simulink model "MC_CVCR_rev6_sim_withc_code_S_function_contplant"  (R2017a)
settings: Solver=VariableStepAuto  StartTime=0.0  StopTime=0.1  FixedStep=T_sim  MaxStep=T_s/10  RelTol=1e-3  EnableMultiTasking=on
model workspace: external: MAT-File C:\Users\Gene\GoogleDrive\UW\Research\Simulation\Discrete CVCR\MATLAB\ws.mat (data not in the file)
values from neighbouring files (symbols this model uses):
  b_a = (-za1*zb1*zc1+1)*J_p/(T_s)    [MC_CVCR_rev6_code_withc_code_S_function.m]
  b_p = 1e-4    (= 0.0001)    [MC_CVCR_rev6_code_withc_code_S_function.m]
  J_p = 6.09e-5    (= 6.09e-05)    [MC_CVCR_rev6_code_withc_code_S_function.m]
  K_i = 2*pi*BW_CVCR*R_s    (= 183.719331443)    [MC_CVCR_rev6_code_withc_code_S_function.m]
  K_isa = ((-(za1+zb1+zc1)+3)*J_p-T_s*b_a-(T_s)^2*K_sa)/((T_s)^3)    [MC_CVCR_rev6_code_withc_code_S_function.m]
  K_p = 2*pi*BW_CVCR*L_s    (= 0.0699004365424)    [MC_CVCR_rev6_code_withc_code_S_function.m]
  K_sa = ((-(za1*zb1+za1*zc1+zb1*zc1)+3)*J_p-2*T_s*b_a)/((T_s)^2)    [MC_CVCR_rev6_code_withc_code_S_function.m]
  K_T = 3/2*K_e    (= 0.013078435501)    [MC_CVCR_rev6_code_withc_code_S_function.m]
  Ksf1 = 1000    [MC_CVCR_rev6_code_withc_code_S_function.m]
  Ksf2 = 4000    [MC_CVCR_rev6_code_withc_code_S_function.m]
  L_ds = 42.28e-6    (= 4.228e-05)    [MC_CVCR_rev6_code_withc_code_S_function.m]
  L_qs = 46.71e-6    (= 4.671e-05)    [MC_CVCR_rev6_code_withc_code_S_function.m]
  Lambda_pm = K_e/(P/2)    (= 0.00217973925016)    [MC_CVCR_rev6_code_withc_code_S_function.m]
  NegSpeedLimit = -600    [MC_CVCR_rev6_code_withc_code_S_function.m]
  P = 8    [MC_CVCR_rev6_code_withc_code_S_function.m]
  PosSpeedLimit = 600    [MC_CVCR_rev6_code_withc_code_S_function.m]
  R_s = 0.116959358962624    (= 0.116959358963)    [MC_CVCR_rev6_code_withc_code_S_function.m]
  T_s = 1/f_s    (= 5e-05)    [MC_CVCR_rev6_code_withc_code_S_function.m]
  T_u = 0.047    [MC_CVCR_rev6_code_withc_code_S_function.m]
libraries: dspsrcs4 x5
settings Model: Creator=Gene  LastModifiedBy=Gene
settings DataIOCC: SaveFormat=StructureWithTime
settings OptimizationCC: LifeSpan=inf
settings DebuggingCC: SFUnexpectedBacktrackingDiag=warning  SFNoUnconditionalDefaultTransitionDiag=warning  SFExecutionAtInitializationDiag=none
settings GRTTargetCC: TargetLangStandard=C89/C90 (ANSI)  GeneratePreprocessorConditionals=Disable all
settings ConfigComp: CovMetricSettings=dw  CovHtmlReporting=on  CovSaveCumulativeToWorkspaceVar=on  CovSaveSingleToWorkspaceVar=on  CovExternalEMLEnable=off

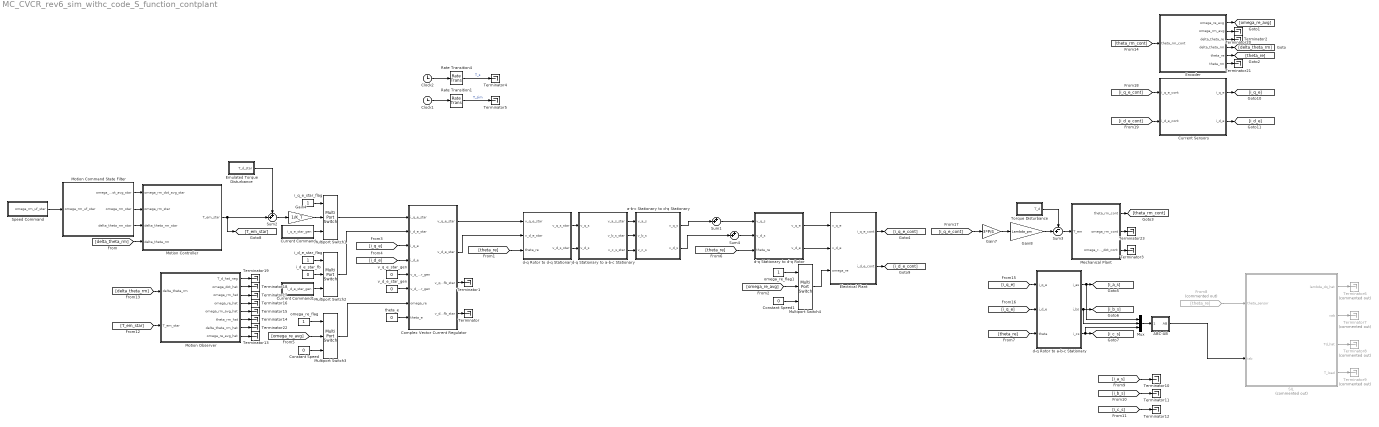
== system MC_CVCR_rev6_sim_withc_code_S_function_contplant ==
  ABC-AB : Subsystem
  Clock1 : Clock
  Clock2 : Clock
  Complex Vector Current Regulator : Subsystem
  Constant Speed : Constant  Value=0  SampleTime=-1
  Constant Speed1 : Constant  Value=0  SampleTime=-1
  Current Command : Subsystem
  Current Command1 : Subsystem
  Current Sensors : Subsystem  TreatAsAtomicUnit=on  SystemSampleTime=T_s
  Electrical Plant : Subsystem
  Emulated Torque Disturbance : Subsystem
  Encoder : Subsystem  TreatAsAtomicUnit=on  SystemSampleTime=T_s
  From8 : From  Commented=on  GotoTag=theta_re
  Gain4 : Gain  Gain=1/K_T
  Gain7 : Gain  Gain=3*P/4
  Gain8 : Gain  Gain=Lambda_pm
  Mechanical Plant : Subsystem
  Motion Command State Filter : Subsystem
  Motion Controller : Subsystem
  Motion Observer : Subsystem
  Multiport Switch{1..4} (4 alike) : MultiPortSwitch  Inputs=2
  Mux : Mux  Inputs=3
  Rate Transition1 : RateTransition  OutPortSampleTime=T_sim
  Rate Transition4 : RateTransition  OutPortSampleTime=T_s
  SIL : Subsystem  Commented=on  TreatAsAtomicUnit=on
  Speed Command : Subsystem
  Sum1 : Sum  Inputs=++|
  Sum2 : Sum  Inputs=++|
  Sum3 : Sum  Inputs=-+|
  Sum4 : Sum  Inputs=++|
  Terminator{,1..5,10..23} (20 alike) : Terminator
  Terminator{6..9} (4 alike) : Terminator  Commented=on
  Torque Disturbance : Subsystem
  a-b-c Stationary to d-q Stationary : Subsystem
  d-q Rotor to d-q Stationary : Subsystem
  d-q Rotor to a-b-c Stationary : Subsystem  TreatAsAtomicUnit=on  SystemSampleTime=T_s
  d-q Stationary to a-b-c Stationary : Subsystem
  d-q Stationary to d-q Rotor : Subsystem
  i_d_e_star_fb : Constant  Value=0  SampleTime=-1
  i_d_e_star_flag : Constant  SampleTime=-1
  i_q_e_star_flag : Constant  SampleTime=-1
  omega_re_flag : Constant  SampleTime=-1
  omega_re_flag1 : Constant  SampleTime=-1
  theta_e : Constant  Value=0
  v_d_e_star_gen : Constant  Value=0
  v_q_e_star_gen : Constant  Value=0
  wires:
  Multiport Switch2/1 -> Complex Vector Current Regulator/2(i_d_e_star)
  Gain4/1 -> Multiport Switch1/2
  Complex Vector Current Regulator/4(v_d_e_sfb_star) -> Terminator/1
  Complex Vector Current Regulator/3(v_q_e_sfb_star) -> Terminator1/1
  v_d_e_star_gen/1 -> Complex Vector Current Regulator/6(v_d_e_star_gen)
  v_q_e_star_gen/1 -> Complex Vector Current Regulator/5(v_q_e_star_gen)
  theta_e/1 -> Complex Vector Current Regulator/8(theta_e)
  Sum2/1 -> Gain4/1
  d-q Stationary to d-q Rotor/1(v_q_e) -> Electrical Plant/1(v_q_e)
  d-q Stationary to d-q Rotor/2(v_d_e) -> Electrical Plant/2(v_d_e)
  Gain7/1 -> Gain8/1
  Gain8/1 -> Sum3/2
  Sum3/1 -> Mechanical Plant/1(T_em)
  Torque Disturbance/1(T_d) -> Sum3/1
  Speed Command/1(omega_rm_uf_star) -> Motion Command State Filter/1(omega_rm_uf_star)
  Emulated Torque Disturbance/1(T_d_star) -> Sum2/1
  Motion Command State Filter/1(omega_rm_dot_avg_star) -> Motion Controller/1(omega_rm_dot_avg_star)
  Motion Command State Filter/2(omega_rm_star) -> Motion Controller/2(omega_rm_star)
  Motion Command State Filter/3(delta_theta_rm_star) -> Motion Controller/3(delta_theta_rm_star)
  Motion Controller/1(T_em_star) -> Sum2/2, [T_em_star]
  [delta_theta_rm] -> Motion Controller/4(delta_theta_rm)
  Multiport Switch4/1 -> Electrical Plant/3(omega_re)
  Multiport Switch3/1 -> Complex Vector Current Regulator/7(omega_re)
  [i_q_e] -> Complex Vector Current Regulator/3(i_q_e)
  [i_d_e] -> Complex Vector Current Regulator/4(i_d_e)
  Clock2/1 -> Rate Transition4/1
  Rate Transition4/1 -> Terminator4/1  "T_s"
  Rate Transition1/1 -> Terminator5/1  "T_sim"
  Clock1/1 -> Rate Transition1/1
  Current Command/1(i_q_e_star_gen) -> Multiport Switch1/3
  i_q_e_star_flag/1 -> Multiport Switch1/1
  Multiport Switch1/1 -> Complex Vector Current Regulator/1(i_q_e_star)
  i_d_e_star_fb/1 -> Multiport Switch2/2
  Current Command1/1(i_d_e_star_gen) -> Multiport Switch2/3
  i_d_e_star_flag/1 -> Multiport Switch2/1
  Constant Speed/1 -> Multiport Switch3/3
  [omega_re_avg] -> Multiport Switch3/2
  omega_re_flag/1 -> Multiport Switch3/1
  Constant Speed1/1 -> Multiport Switch4/3
  omega_re_flag1/1 -> Multiport Switch4/1
  [omega_re_avg] -> Multiport Switch4/2
  d-q Rotor to d-q Stationary/1(v_q_s_star) -> d-q Stationary to a-b-c Stationary/1(v_q_s)
  d-q Rotor to d-q Stationary/2(v_d_s_star) -> d-q Stationary to a-b-c Stationary/2(v_d_s)
  Sum1/1 -> d-q Stationary to d-q Rotor/1(v_q_s)
  Sum4/1 -> d-q Stationary to d-q Rotor/2(v_d_s)
  d-q Stationary to a-b-c Stationary/1(v_a_s_star) -> a-b-c Stationary to d-q Stationary/1(v_a_s)
  d-q Stationary to a-b-c Stationary/2(v_b_s_star) -> a-b-c Stationary to d-q Stationary/2(v_b_s)
  d-q Stationary to a-b-c Stationary/3(v_c_s_star) -> a-b-c Stationary to d-q Stationary/3(v_c_s)
  [theta_re] -> d-q Rotor to d-q Stationary/3(theta_re)
  [theta_re] -> d-q Stationary to d-q Rotor/3(theta_re)
  Complex Vector Current Regulator/2(v_d_e_star) -> d-q Rotor to d-q Stationary/2(v_d_e_star)
  Complex Vector Current Regulator/1(v_q_e_star) -> d-q Rotor to d-q Stationary/1(v_q_e_star)
  [theta_re] -> d-q Rotor to a-b-c Stationary/3(theta)
  Mux/1 -> ABC-AB/1(ABC)
  d-q Rotor to a-b-c Stationary/3(i_cs) -> Mux/3, [i_c_s]
  d-q Rotor to a-b-c Stationary/2(i_bs) -> Mux/2, [i_b_s]
  d-q Rotor to a-b-c Stationary/1(i_as) -> Mux/1, [i_a_s]
  From8/1 -> SIL/1(theta_sensor)
  ABC-AB/1(AB) -> SIL/2(iab)
  SIL/1(lambda_dq_hat) -> Terminator6/1
  SIL/2(vab) -> Terminator7/1
  SIL/3(Td_hat) -> Terminator8/1
  SIL/4(T_load) -> Terminator9/1
  [i_a_s] -> Terminator10/1
  [i_b_s] -> Terminator11/1
  [i_c_s] -> Terminator12/1
  [delta_theta_rm] -> Motion Observer/1(delta_theta_rm)
  [T_em_star] -> Motion Observer/2(T_em_star)
  Motion Observer/7(delta_theta_rm_hat) -> Terminator22/1
  Motion Observer/6(theta_rm_hat) -> Terminator14/1
  Motion Observer/5(omega_rm_avg_hat) -> Terminator15/1
  Motion Observer/4(omega_re_hat) -> Terminator16/1
  Motion Observer/3(omega_rm_hat) -> Terminator17/1
  Motion Observer/2(omega_dot_hat) -> Terminator18/1
  Motion Observer/1(T_d_hat_neg) -> Terminator19/1
  Motion Observer/8(omega_re_avg_hat) -> Terminator13/1
  a-b-c Stationary to d-q Stationary/1(v_q_s) -> Sum1/2
  a-b-c Stationary to d-q Stationary/2(v_d_s) -> Sum4/2
  [i_q_e] -> d-q Rotor to a-b-c Stationary/2(i_d_e)
  Encoder/4(delta_theta_rm) -> [delta_theta_rm]
  Encoder/2(omega_rm_avg) -> Terminator20/1
  Encoder/6(theta_rm) -> Terminator21/1
  Encoder/1(omega_re_avg) -> [omega_re_avg]
  Encoder/5(theta_re) -> [theta_re]
  Encoder/3(delta_theta_re) -> Terminator2/1
  Mechanical Plant/3(omega_rm_dot_cont) -> Terminator3/1
  Mechanical Plant/2(omega_rm_cont) -> Terminator23/1
  Mechanical Plant/1(theta_rm_cont) -> [theta_rm_cont]
  [theta_rm_cont] -> Encoder/1(theta_rm_cont)
  Electrical Plant/2(i_d_e_cont) -> [i_d_e_cont]
  Electrical Plant/1(i_q_e_cont) -> [i_q_e_cont]
  [i_q_e] -> d-q Rotor to a-b-c Stationary/1(i_q_e)
  [i_q_e_cont] -> Gain7/1
  [i_d_e_cont] -> Current Sensors/2(i_d_e_cont)
  [i_q_e_cont] -> Current Sensors/1(i_q_e_cont)
  Current Sensors/1(i_q_e) -> [i_q_e]
  Current Sensors/2(i_d_e) -> [i_d_e]

== system MC_CVCR_rev6_sim_withc_code_S_function_contplant/ABC-AB ==
  ABC : Inport
  Mux2 : Mux  Inputs=2
  a : Fcn  Expr=2/3*(u[1] -0.5*u[2] - 0.5*u[3])
  b : Fcn  Expr=2/3*(0 +sqrt(3)/2*u[2] - sqrt(3)/2*u[3])
  AB : Outport
  wires:
  Mux2/1 -> AB/1
  b/1 -> Mux2/2
  ABC/1 -> b/1, a/1
  a/1 -> Mux2/1

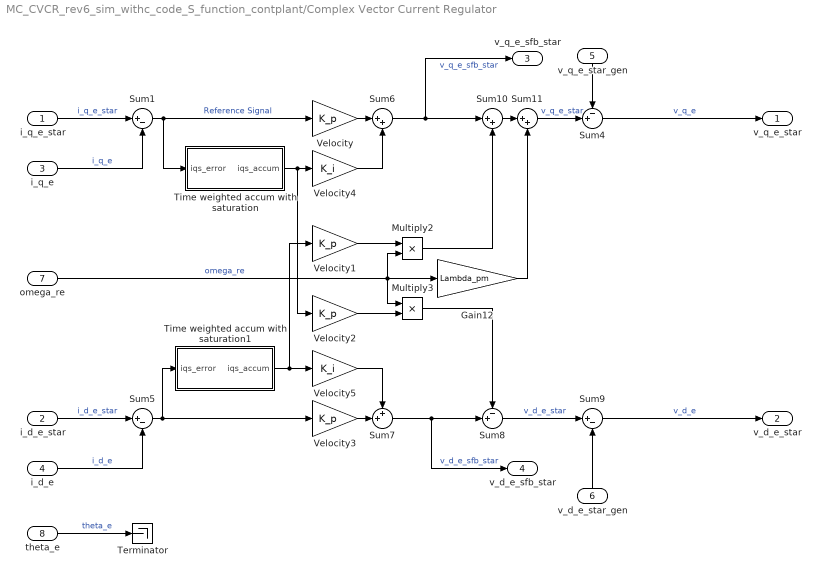
== system MC_CVCR_rev6_sim_withc_code_S_function_contplant/Complex Vector Current Regulator ==
  i_q_e_star : Inport
  i_d_e_star : Inport  Port=2
  i_q_e : Inport  Port=3
  i_d_e : Inport  Port=4
  v_q_e_star_gen : Inport  Port=5
  v_d_e_star_gen : Inport  Port=6
  omega_re : Inport  Port=7
  theta_e : Inport  Port=8
  Gain12 : Gain  Gain=Lambda_pm
  Multiply2 : Product  Inputs=**
  Multiply3 : Product  Inputs=**
  Sum1 : Sum  Priority=1  Inputs=|+-
  Sum10 : Sum  Priority=1  Inputs=|++
  Sum11 : Sum  Priority=1  Inputs=|++
  Sum4 : Sum  Priority=1  Inputs=-+|
  Sum5 : Sum  Priority=1  Inputs=|+-
  Sum6 : Sum  Priority=1  Inputs=|++
  Sum7 : Sum  Priority=1  Inputs=++|
  Sum8 : Sum  Priority=1  Inputs=-+|
  Sum9 : Sum  Inputs=|+-
  Terminator : Terminator
  Time weighted accum with saturation : Subsystem
  Time weighted accum with saturation1 : Subsystem
  Velocity{,1..3} (4 alike) : Gain  Gain=K_p  SampleTime=T_s
  Velocity4 : Gain  Gain=K_i  SampleTime=T_s
  Velocity5 : Gain  Gain=K_i  SampleTime=T_s
  v_q_e_star : Outport
  v_d_e_star : Outport  Port=2
  v_q_e_sfb_star : Outport  Port=3
  v_d_e_sfb_star : Outport  Port=4
  wires:
  Velocity2/1 -> Multiply3/2
  Sum1/1 -> Velocity/1, Time weighted accum with saturation/1(iqs_error)  "Reference Signal"
  i_q_e_star/1 -> Sum1/1  "i_q_e_star"
  i_d_e_star/1 -> Sum5/1  "i_d_e_star"
  Time weighted accum with saturation/1(iqs_accum) -> Velocity4/1, Velocity2/1
  Sum5/1 -> Time weighted accum with saturation1/1(iqs_error), Velocity3/1
  Time weighted accum with saturation1/1(iqs_accum) -> Velocity5/1, Velocity1/1
  Velocity4/1 -> Sum6/2
  Velocity/1 -> Sum6/1
  Velocity3/1 -> Sum7/2
  Velocity5/1 -> Sum7/1
  Sum7/1 -> v_d_e_sfb_star/1, Sum8/2  "v_d_e_sfb_star"
  Sum6/1 -> v_q_e_sfb_star/1, Sum10/1  "v_q_e_sfb_star"
  Multiply3/1 -> Sum8/1
  Multiply2/1 -> Sum10/2
  Sum11/1 -> Sum4/2  "v_q_e_star"
  Sum10/1 -> Sum11/1
  Gain12/1 -> Sum11/2
  Sum8/1 -> Sum9/1  "v_d_e_star"
  v_q_e_star_gen/1 -> Sum4/1
  Velocity1/1 -> Multiply2/1
  omega_re/1 -> Multiply3/1, Gain12/1, Multiply2/2  "omega_re"
  v_d_e_star_gen/1 -> Sum9/2
  theta_e/1 -> Terminator/1  "theta_e"
  Sum4/1 -> v_q_e_star/1  "v_q_e"
  Sum9/1 -> v_d_e_star/1  "v_d_e"
  i_q_e/1 -> Sum1/2  "i_q_e"
  i_d_e/1 -> Sum5/2  "i_d_e"

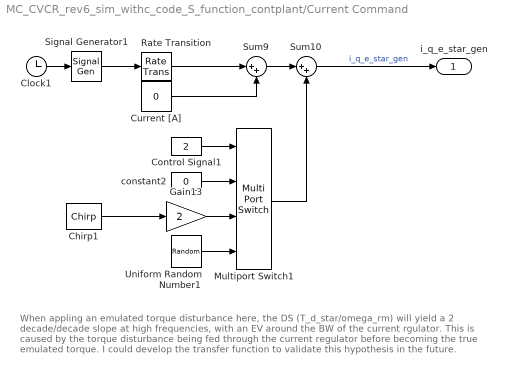
== system MC_CVCR_rev6_sim_withc_code_S_function_contplant/Current Command ==
  note: When appling an emulated torque disturbance here, the DS (T_d_star/omega_rm) will yield
      | a 2 decade/decade slope at high frequencies, with an EV around the BW of the current rgulator.
      | This is caused by the torque disturbance being fed through the current regulator before becoming the true emulated torque.
      |
      | I could develop the transfer function to validate this hypothesis in the future.
  Chirp1 : dspsrcs4/Chirp  sweep=Logarithmic  mode=Bidirectional  f0=0.1  f1=1000  t1=2  Tsweep=2  phase=0  Ts=T_s  spf=1  datatype=Double  OutputFrames=on
      settings: SourceProductName=DSP System Toolbox
  Clock1 : Clock
  Control Signal1 : Constant  Value=2
  Current [A] : Constant  Value=0
  Gain13 : Gain  Gain=2
  Multiport Switch1 : MultiPortSwitch
  Rate Transition : RateTransition  OutPortSampleTime=T_s
  Signal Generator1 : SignalGenerator  TimeSource=Use external signal  Amplitude=0
  Sum10 : Sum  Inputs=|++
  Sum9 : Sum  Inputs=|++
  Uniform Random Number1 : UniformRandomNumber  Minimum=-0.1  Maximum=0.1  SampleTime=T_s
  constant2 : Constant  Value=0
  i_q_e_star_gen : Outport
  wires:
  Multiport Switch1/1 -> Sum10/2
  Chirp1/1 -> Gain13/1
  Uniform Random Number1/1 -> Multiport Switch1/4
  Current [A]/1 -> Sum9/2
  Signal Generator1/1 -> Rate Transition/1
  Control Signal1/1 -> Multiport Switch1/1
  Clock1/1 -> Signal Generator1/1
  constant2/1 -> Multiport Switch1/2
  Sum9/1 -> Sum10/1
  Gain13/1 -> Multiport Switch1/3
  Sum10/1 -> i_q_e_star_gen/1  "i_q_e_star_gen"
  Rate Transition/1 -> Sum9/1

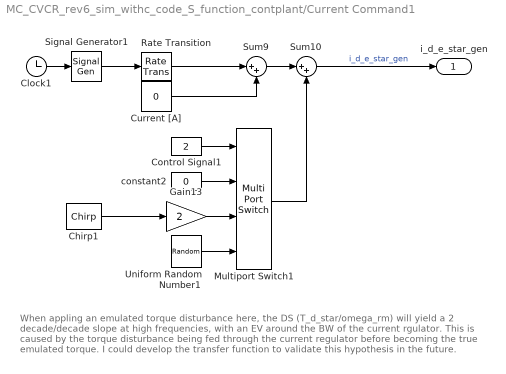
== system MC_CVCR_rev6_sim_withc_code_S_function_contplant/Current Command1 ==
  note: When appling an emulated torque disturbance here, the DS (T_d_star/omega_rm) will yield
      | a 2 decade/decade slope at high frequencies, with an EV around the BW of the current rgulator.
      | This is caused by the torque disturbance being fed through the current regulator before becoming the true emulated torque.
      |
      | I could develop the transfer function to validate this hypothesis in the future.
  Chirp1 : dspsrcs4/Chirp  sweep=Logarithmic  mode=Bidirectional  f0=0.1  f1=1000  t1=2  Tsweep=2  phase=0  Ts=T_s  spf=1  datatype=Double  OutputFrames=on
      settings: SourceProductName=DSP System Toolbox
  Clock1 : Clock
  Control Signal1 : Constant  Value=2
  Current [A] : Constant  Value=0
  Gain13 : Gain  Gain=2
  Multiport Switch1 : MultiPortSwitch
  Rate Transition : RateTransition  OutPortSampleTime=T_s
  Signal Generator1 : SignalGenerator  TimeSource=Use external signal  Amplitude=0
  Sum10 : Sum  Inputs=|++
  Sum9 : Sum  Inputs=|++
  Uniform Random Number1 : UniformRandomNumber  Minimum=-0.1  Maximum=0.1  SampleTime=T_s
  constant2 : Constant  Value=0
  i_d_e_star_gen : Outport
  wires:
  Multiport Switch1/1 -> Sum10/2
  Chirp1/1 -> Gain13/1
  Uniform Random Number1/1 -> Multiport Switch1/4
  Current [A]/1 -> Sum9/2
  Signal Generator1/1 -> Rate Transition/1
  Control Signal1/1 -> Multiport Switch1/1
  Clock1/1 -> Signal Generator1/1
  constant2/1 -> Multiport Switch1/2
  Sum9/1 -> Sum10/1
  Gain13/1 -> Multiport Switch1/3
  Sum10/1 -> i_d_e_star_gen/1  "i_d_e_star_gen"
  Rate Transition/1 -> Sum9/1

== system MC_CVCR_rev6_sim_withc_code_S_function_contplant/Current Sensors ==
  i_q_e_cont : Inport
  i_d_e_cont : Inport  Port=2
  i_q_e : Outport
  i_d_e : Outport  Port=2
  wires:
  i_q_e_cont/1 -> i_q_e/1  "i_q_e"
  i_d_e_cont/1 -> i_d_e/1  "i_q_e"

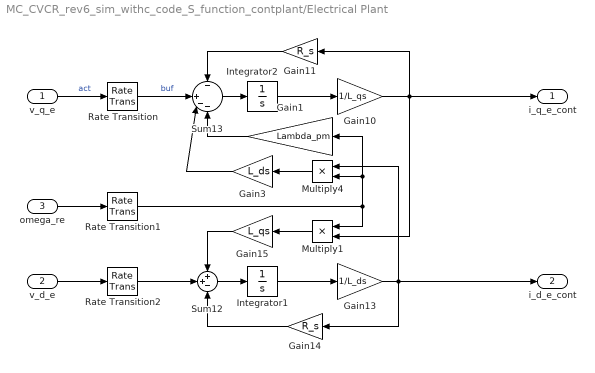
== system MC_CVCR_rev6_sim_withc_code_S_function_contplant/Electrical Plant ==
  v_q_e : Inport
  v_d_e : Inport  Port=2
  omega_re : Inport  Port=3
  Gain1 : Gain  Gain=Lambda_pm
  Gain10 : Gain  Gain=1/L_qs
  Gain11 : Gain  Gain=R_s
  Gain13 : Gain  Gain=1/L_ds
  Gain14 : Gain  Gain=R_s
  Gain15 : Gain  Gain=L_qs
  Gain3 : Gain  Gain=L_ds
  Integrator1 : Integrator
  Integrator2 : Integrator
  Multiply1 : Product  Inputs=**
  Multiply4 : Product  Inputs=**
  Rate Transition : RateTransition
  Rate Transition1 : RateTransition
  Rate Transition2 : RateTransition
  Sum12 : Sum  Inputs=++-
  Sum13 : Sum  Inputs=-|+--
  i_q_e_cont : Outport
  i_d_e_cont : Outport  Port=2
  wires:
  v_d_e/1 -> Rate Transition2/1
  v_q_e/1 -> Rate Transition/1  "act"
  Integrator1/1 -> Gain13/1
  Gain13/1 -> i_d_e_cont/1, Gain14/1, Multiply4/1
  Sum12/1 -> Integrator1/1
  Integrator2/1 -> Gain10/1
  Gain10/1 -> Multiply1/2, i_q_e_cont/1, Gain11/1
  Sum13/1 -> Integrator2/1
  Gain3/1 -> Sum13/3
  Gain15/1 -> Sum12/1
  Gain14/1 -> Sum12/3
  Gain11/1 -> Sum13/1
  Multiply1/1 -> Gain15/1
  Multiply4/1 -> Gain3/1
  omega_re/1 -> Rate Transition1/1
  Gain1/1 -> Sum13/4
  Rate Transition/1 -> Sum13/2  "buf"
  Rate Transition1/1 -> Multiply1/1, Gain1/1, Multiply4/2
  Rate Transition2/1 -> Sum12/2

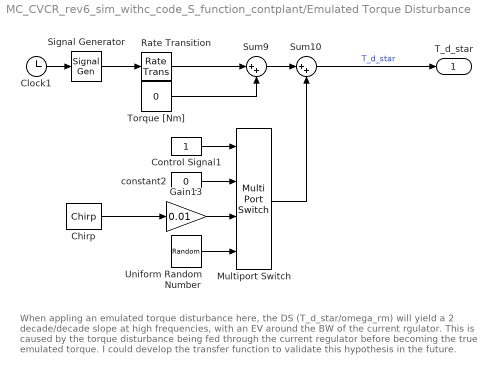
== system MC_CVCR_rev6_sim_withc_code_S_function_contplant/Emulated Torque Disturbance ==
  note: When appling an emulated torque disturbance here, the DS (T_d_star/omega_rm) will yield
      | a 2 decade/decade slope at high frequencies, with an EV around the BW of the current rgulator.
      | This is caused by the torque disturbance being fed through the current regulator before becoming the true emulated torque.
      |
      | I could develop the transfer function to validate this hypothesis in the future.
  Chirp : dspsrcs4/Chirp  sweep=Logarithmic  mode=Bidirectional  f0=0.1  f1=250  t1=5  Tsweep=5  phase=0  Ts=T_s  spf=1  datatype=Double  OutputFrames=on
      settings: SourceProductName=DSP System Toolbox
  Clock1 : Clock
  Control Signal1 : Constant
  Gain13 : Gain  Gain=0.01
  Multiport Switch : MultiPortSwitch
  Rate Transition : RateTransition  OutPortSampleTime=T_s
  Signal Generator : SignalGenerator  TimeSource=Use external signal  Amplitude=0
  Sum10 : Sum  Inputs=|++
  Sum9 : Sum  Inputs=|++
  Torque [Nm] : Constant  Value=0
  Uniform Random Number : UniformRandomNumber  Minimum=-0.1  Maximum=0.1  SampleTime=T_s
  constant2 : Constant  Value=0
  T_d_star : Outport
  wires:
  Multiport Switch/1 -> Sum10/2
  Chirp/1 -> Gain13/1
  Uniform Random Number/1 -> Multiport Switch/4
  Torque [Nm]/1 -> Sum9/2
  Signal Generator/1 -> Rate Transition/1
  Control Signal1/1 -> Multiport Switch/1
  Clock1/1 -> Signal Generator/1
  constant2/1 -> Multiport Switch/2
  Sum9/1 -> Sum10/1
  Gain13/1 -> Multiport Switch/3
  Sum10/1 -> T_d_star/1  "T_d_star"
  Rate Transition/1 -> Sum9/1

== system MC_CVCR_rev6_sim_withc_code_S_function_contplant/Encoder ==
  theta_rm_cont : Inport
  Discrete Transfer Fcn : DiscreteTransferFcn  Numerator=[1 -1]  Denominator=[1 0]
  Gain1 : Gain  Gain=P/2
  Gain2 : Gain  Gain=P/2
  Gain3 : Gain  Gain=P/2
  Gain5 : Gain  Gain=1/T_s
  omega_re_avg : Outport
  omega_rm_avg : Outport  Port=2
  delta_theta_re : Outport  Port=3
  delta_theta_rm : Outport  Port=4
  theta_re : Outport  Port=5
  theta_rm : Outport  Port=6
  wires:
  theta_rm_cont/1 -> theta_rm/1, Gain1/1, Discrete Transfer Fcn/1  "theta_rm"
  Discrete Transfer Fcn/1 -> delta_theta_rm/1, Gain3/1, Gain5/1  "delta_theta_rm"
  Gain5/1 -> omega_rm_avg/1, Gain2/1  "omega_rm_avg"
  Gain1/1 -> theta_re/1  "theta_re"
  Gain2/1 -> omega_re_avg/1  "omega_re_avg"
  Gain3/1 -> delta_theta_re/1  "delta_theta_re"

== system MC_CVCR_rev6_sim_withc_code_S_function_contplant/Mechanical Plant ==
  T_em : Inport
  Gain : Gain  Gain=1/J_p
  Gain1 : Gain  Gain=T_u
  Gain12 : Gain  Gain=b_p
  Integrator2 : Integrator
  Integrator3 : Integrator
  Sign : Signum  ZeroCross=off
  Sum11 : Sum  Inputs=||+--
  theta_rm_cont : Outport
  omega_rm_cont : Outport  Port=2
  omega_rm_dot_cont : Outport  Port=3
  wires:
  Gain/1 -> omega_rm_dot_cont/1, Integrator2/1  "omega_rm_dot"
  Sign/1 -> Gain1/1
  Sum11/1 -> Gain/1
  Integrator2/1 -> omega_rm_cont/1, Integrator3/1, Gain12/1, Sign/1  "omega_rm"
  Integrator3/1 -> theta_rm_cont/1  "theta_re"
  Gain12/1 -> Sum11/3  "T_bp"
  T_em/1 -> Sum11/1  "T_em"
  Gain1/1 -> Sum11/2  "T_u"

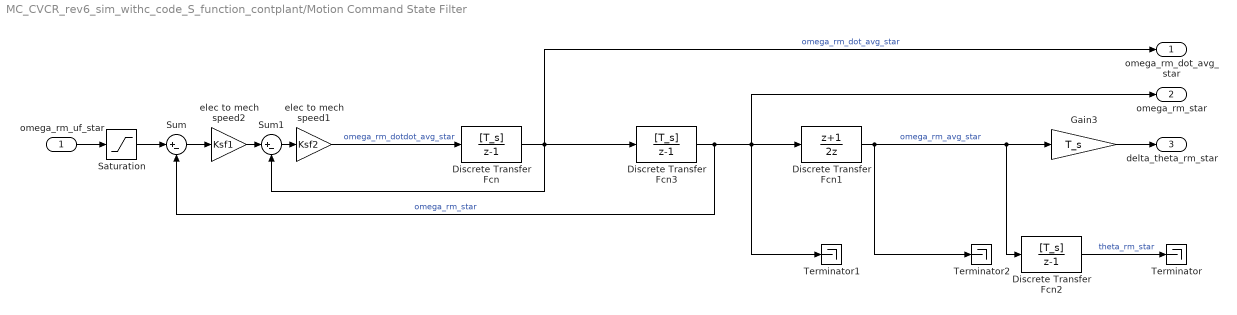
== system MC_CVCR_rev6_sim_withc_code_S_function_contplant/Motion Command State Filter ==
  omega_rm_uf_star : Inport
  " elec to mech speed1" : Gain  Gain=Ksf2
  " elec to mech speed2" : Gain  Gain=Ksf1
  Discrete Transfer Fcn : DiscreteTransferFcn  Numerator=[T_s]  Denominator=[1 -1]
  Discrete Transfer Fcn1 : DiscreteTransferFcn  Numerator=[1 1]  Denominator=[2 0]
  Discrete Transfer Fcn2 : DiscreteTransferFcn  Numerator=[T_s]  Denominator=[1 -1]
  Discrete Transfer Fcn3 : DiscreteTransferFcn  Numerator=[T_s]  Denominator=[1 -1]
  Gain3 : Gain  Gain=T_s
  Saturation : Saturate  UpperLimit=PosSpeedLimit  LowerLimit=NegSpeedLimit
  Sum : Sum  Inputs=|+-
  Sum1 : Sum  Inputs=|+-
  Terminator : Terminator
  Terminator1 : Terminator
  Terminator2 : Terminator
  omega_rm_dot_avg_star : Outport
  omega_rm_star : Outport  Port=2
  delta_theta_rm_star : Outport  Port=3
  wires:
  Sum/1 -> " elec to mech speed2"/1
  Discrete Transfer Fcn1/1 -> Gain3/1, Discrete Transfer Fcn2/1, Terminator2/1  "omega_rm_avg_star"
  omega_rm_uf_star/1 -> Saturation/1
  Discrete Transfer Fcn/1 -> Discrete Transfer Fcn3/1, omega_rm_dot_avg_star/1, Sum1/2  "omega_rm_dot_avg_star"
  Discrete Transfer Fcn2/1 -> Terminator/1  "theta_rm_star"
  " elec to mech speed2"/1 -> Sum1/1
  Sum1/1 -> " elec to mech speed1"/1
  " elec to mech speed1"/1 -> Discrete Transfer Fcn/1  "omega_rm_dotdot_avg_star"
  Discrete Transfer Fcn3/1 -> Sum/2, omega_rm_star/1, Discrete Transfer Fcn1/1, Terminator1/1  "omega_rm_star"
  Gain3/1 -> delta_theta_rm_star/1
  Saturation/1 -> Sum/1

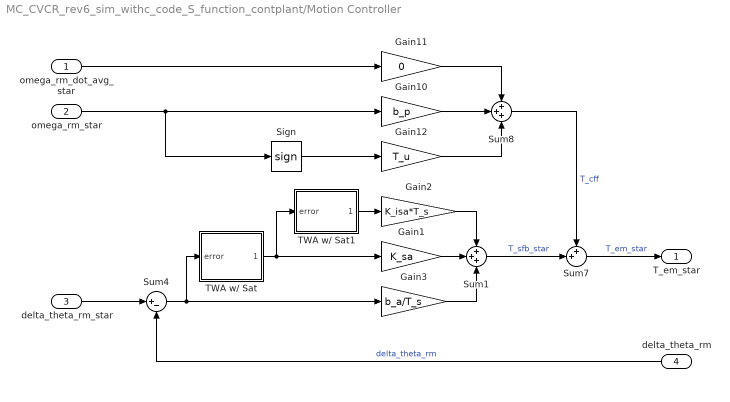
== system MC_CVCR_rev6_sim_withc_code_S_function_contplant/Motion Controller ==
  omega_rm_dot_avg_star : Inport
  omega_rm_star : Inport  Port=2
  delta_theta_rm_star : Inport  Port=3
  delta_theta_rm : Inport  Port=4
  Gain1 : Gain  Gain=K_sa
  Gain10 : Gain  Gain=b_p
  Gain11 : Gain  Gain=0
  Gain12 : Gain  Gain=T_u
  Gain2 : Gain  Gain=K_isa*T_s
  Gain3 : Gain  Gain=b_a/T_s
  Sign : Signum  ZeroCross=off
  Sum1 : Sum  Inputs=+++
  Sum4 : Sum  Inputs=|+-
  Sum7 : Sum  Inputs=++|
  Sum8 : Sum  Inputs=+++
  TWA w/ Sat : Subsystem
  TWA w/ Sat1 : Subsystem
  T_em_star : Outport
  wires:
  Gain2/1 -> Sum1/1
  Gain3/1 -> Sum1/3
  Gain1/1 -> Sum1/2
  Sum4/1 -> TWA w/ Sat/1(error), Gain3/1
  Sum7/1 -> T_em_star/1  "T_em_star"
  TWA w/ Sat/1(accum) -> TWA w/ Sat1/1(error), Gain1/1
  TWA w/ Sat1/1(accum) -> Gain2/1
  delta_theta_rm_star/1 -> Sum4/1
  Sum1/1 -> Sum7/2  "T_sfb_star"
  omega_rm_dot_avg_star/1 -> Gain11/1
  omega_rm_star/1 -> Sign/1, Gain10/1
  Sign/1 -> Gain12/1
  Gain12/1 -> Sum8/3
  Gain10/1 -> Sum8/2
  Gain11/1 -> Sum8/1
  Sum8/1 -> Sum7/1  "T_cff"
  delta_theta_rm/1 -> Sum4/2  "delta_theta_rm"

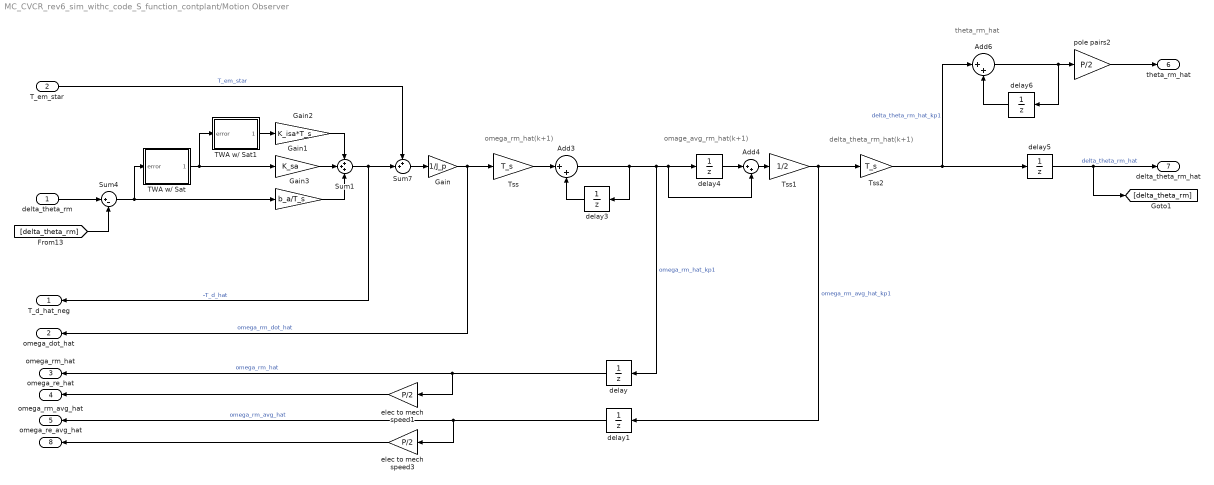
== system MC_CVCR_rev6_sim_withc_code_S_function_contplant/Motion Observer ==
  note: omega_rm_hat(k+1)
  note: delta_theta_rm_hat(k+1)
  note: omage_avg_rm_hat(k+1)
  note: theta_rm_hat
  delta_theta_rm : Inport
  T_em_star : Inport  Port=2
  " elec to mech speed1" : Gain  Gain=P/2
  " elec to mech speed3" : Gain  Gain=P/2
  Add3 : Sum  Inputs=|++
  Add4 : Sum  Inputs=|++
  Add6 : Sum  Inputs=|++
  Gain : Gain  Gain=1/J_p
  Gain1 : Gain  Gain=K_sa
  Gain2 : Gain  Gain=K_isa*T_s
  Gain3 : Gain  Gain=b_a/T_s
  Sum1 : Sum  Inputs=+++
  Sum4 : Sum  Inputs=|+-
  Sum7 : Sum  Inputs=++|
  TWA w/ Sat : Subsystem
  TWA w/ Sat1 : Subsystem
  Tss : Gain  Gain=T_s
  Tss1 : Gain  Gain=1/2
  Tss2 : Gain  Gain=T_s
  delay{,1,3..6} (6 alike) : UnitDelay  SampleTime=-1
  pole pairs2 : Gain  Gain=P/2
  T_d_hat_neg : Outport
  omega_dot_hat : Outport  Port=2
  omega_rm_hat : Outport  Port=3
  omega_re_hat : Outport  Port=4
  omega_rm_avg_hat : Outport  Port=5
  theta_rm_hat : Outport  Port=6
  delta_theta_rm_hat : Outport  Port=7
  omega_re_avg_hat : Outport  Port=8
  wires:
  Gain2/1 -> Sum1/1
  Gain3/1 -> Sum1/3
  Gain1/1 -> Sum1/2
  Sum4/1 -> TWA w/ Sat/1(error), Gain3/1
  Sum7/1 -> Gain/1
  TWA w/ Sat/1(accum) -> TWA w/ Sat1/1(error), Gain1/1
  TWA w/ Sat1/1(accum) -> Gain2/1
  delta_theta_rm/1 -> Sum4/1
  Sum1/1 -> Sum7/2, T_d_hat_neg/1  "-T_d_hat"
  T_em_star/1 -> Sum7/1  "T_em_star"
  delay6/1 -> Add6/2
  delay4/1 -> Add4/1
  delay5/1 -> [delta_theta_rm], delta_theta_rm_hat/1  "delta_theta_rm_hat"
  " elec to mech speed1"/1 -> omega_re_hat/1
  Tss1/1 -> Tss2/1, delay1/1  "omega_rm_avg_hat_kp1"
  delay3/1 -> Add3/2
  pole pairs2/1 -> theta_rm_hat/1
  Add6/1 -> delay6/1, pole pairs2/1
  Add4/1 -> Tss1/1
  Tss2/1 -> Add6/1, delay5/1  "delta_theta_rm_hat_kp1"
  Tss/1 -> Add3/1
  " elec to mech speed3"/1 -> omega_re_avg_hat/1
  Gain/1 -> Tss/1, omega_dot_hat/1  "omega_rm_dot_hat"
  Add3/1 -> delay/1, Add4/2, delay4/1, delay3/1  "omega_rm_hat_kp1"
  [delta_theta_rm] -> Sum4/2
  delay/1 -> " elec to mech speed1"/1, omega_rm_hat/1  "omega_rm_hat"
  delay1/1 -> " elec to mech speed3"/1, omega_rm_avg_hat/1  "omega_rm_avg_hat"

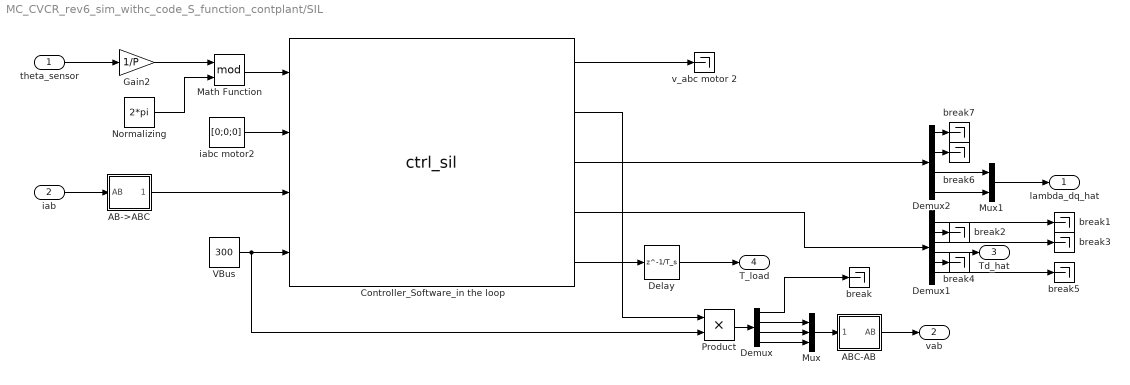
== system MC_CVCR_rev6_sim_withc_code_S_function_contplant/SIL ==
  theta_sensor : Inport
  iab : Inport  Port=2
  AB->ABC : Subsystem
  ABC-AB : Subsystem
  Controller_Software_in the loop : S-Function  FunctionName=ctrl_sil  Parameters=wr_set, T_com_set, lambda_com_set  SFunctionDeploymentMode=off  EnableBusSupport=off  mask{wr_set=20, T_com_set=0, lambda_com_set=Lambda_pm}
      mask prompts: wr_set "Speed"; T_com_set "Torque"; lambda_com_set "Flux"
      mask Display:
      | image('governor.png')
      | port_label('output', 1, 'v_abc_motor2');
      | port_label('output', 2, 'v_abc_motor1');
      | port_label('output', 3, 'Current & Flux');
      | port_label('output', 4, 'debug');
      | port_label('output', 5, 'T_load');
  Delay : Delay  DelayLength=1/T_s
  Demux : Demux
  Demux1 : Demux  Outputs=6
  Demux2 : Demux
  Gain2 : Gain  Gain=1/P
  Math Function : Math  Operator=mod  SampleTime=T_s  SaturateOnIntegerOverflow=on
  Mux : Mux  Inputs=3
  Mux1 : Mux  Inputs=2
  Normalizing : Constant  Value=2*pi  SampleTime=T_s
  Product : Product
  VBus : Constant  Value=300  SampleTime=T_s
  break{,1..7} (8 alike) : Terminator
  iabc motor2 : Constant  Value=[0;0;0]  SampleTime=T_s
  v_abc motor 2 : Terminator
  lambda_dq_hat : Outport
  vab : Outport  Port=2
  Td_hat : Outport  Port=3
  T_load : Outport  Port=4
  wires:
  theta_sensor/1 -> Gain2/1
  Controller_Software_in the loop/2 -> Product/1
  VBus/1 -> Product/2, Controller_Software_in the loop/4
  AB->ABC/1(ABC) -> Controller_Software_in the loop/3
  Normalizing/1 -> Math Function/2
  Math Function/1 -> Controller_Software_in the loop/1
  Controller_Software_in the loop/4 -> Demux1/1
  Controller_Software_in the loop/1 -> v_abc motor 2/1
  iab/1 -> AB->ABC/1(AB)
  iabc motor2/1 -> Controller_Software_in the loop/2
  Gain2/1 -> Math Function/1
  Demux/2 -> Mux/1
  Demux/3 -> Mux/2
  Demux/4 -> Mux/3
  Demux/1 -> break/1
  Product/1 -> Demux/1
  Controller_Software_in the loop/5 -> Delay/1
  Delay/1 -> T_load/1
  Demux1/4 -> Td_hat/1
  Controller_Software_in the loop/3 -> Demux2/1
  Demux2/4 -> Mux1/2
  Demux2/3 -> Mux1/1
  Mux1/1 -> lambda_dq_hat/1
  Mux/1 -> ABC-AB/1(ABC)
  ABC-AB/1(AB) -> vab/1
  Demux1/1 -> break1/1
  Demux1/2 -> break2/1
  Demux1/3 -> break3/1
  Demux1/5 -> break4/1
  Demux1/6 -> break5/1
  Demux2/2 -> break6/1
  Demux2/1 -> break7/1

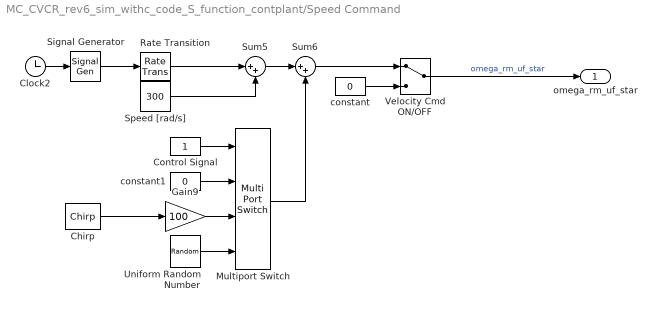
== system MC_CVCR_rev6_sim_withc_code_S_function_contplant/Speed Command ==
  Chirp : dspsrcs4/Chirp  sweep=Linear  mode=Bidirectional  f0=0.001  f1=100  t1=2  Tsweep=2  phase=0  Ts=T_s  spf=1  datatype=Double  OutputFrames=on
      settings: SourceProductName=DSP System Toolbox
  Clock2 : Clock
  Control Signal : Constant
  Gain9 : Gain  Gain=100
  Multiport Switch : MultiPortSwitch
  Rate Transition : RateTransition  OutPortSampleTime=T_s
  Signal Generator : SignalGenerator  TimeSource=Use external signal  Amplitude=0  Frequency=5
  Speed [rad/s] : Constant  Value=300
  Sum5 : Sum  Inputs=|++
  Sum6 : Sum  Inputs=|++
  Uniform Random Number : UniformRandomNumber  Minimum=-50  Maximum=50  SampleTime=T_s
  Velocity Cmd ON/OFF : ManualSwitch
  constant : Constant  Value=0
  constant1 : Constant  Value=0
  omega_rm_uf_star : Outport
  wires:
  Sum5/1 -> Sum6/1
  constant/1 -> Velocity Cmd ON/OFF/2
  Clock2/1 -> Signal Generator/1
  Speed [rad/s]/1 -> Sum5/2
  Signal Generator/1 -> Rate Transition/1
  constant1/1 -> Multiport Switch/2
  Chirp/1 -> Gain9/1
  Uniform Random Number/1 -> Multiport Switch/4
  Control Signal/1 -> Multiport Switch/1
  Multiport Switch/1 -> Sum6/2
  Sum6/1 -> Velocity Cmd ON/OFF/1
  Velocity Cmd ON/OFF/1 -> omega_rm_uf_star/1  "omega_rm_uf_star"
  Gain9/1 -> Multiport Switch/3
  Rate Transition/1 -> Sum5/1

== system MC_CVCR_rev6_sim_withc_code_S_function_contplant/Torque Disturbance ==
  note: Note: Inject Random Noise, sampled at T_s (not T_sim)
      | because yields better DS plots (better coherence),
      | note that T_sim is more realistic though!
  note: Have verified b_a and J_p asymptotes on DS FRF.
  note: only for logging at T_s, so can do DS plots
  Chirp : dspsrcs4/Chirp  sweep=Logarithmic  mode=Bidirectional  f0=0.1  f1=50  t1=5  Tsweep=5  phase=0  Ts=T_s  spf=1  datatype=Single  OutputFrames=on
      settings: SourceProductName=DSP System Toolbox
  Clock1 : Clock
  Control Signal1 : Constant  Value=2
  Gain13 : Gain  Gain=0.1
  Multiport Switch : MultiPortSwitch
  Rate Transition : RateTransition  OutPortSampleTime=T_s
  Signal Generator : SignalGenerator  TimeSource=Use external signal  Amplitude=0  Frequency=100
  Sum10 : Sum  Inputs=|++
  Sum9 : Sum  Inputs=|++
  Torque [Nm] : Constant  Value=0
  Uniform Random Number : UniformRandomNumber  Minimum=-0.1  Maximum=0.1  SampleTime=T_s
  constant2 : Constant  Value=0
  T_d : Outport
  wires:
  Multiport Switch/1 -> Sum10/2
  Chirp/1 -> Gain13/1
  Uniform Random Number/1 -> Multiport Switch/4
  Torque [Nm]/1 -> Sum9/2
  Signal Generator/1 -> Rate Transition/1
  Control Signal1/1 -> Multiport Switch/1
  Clock1/1 -> Signal Generator/1
  constant2/1 -> Multiport Switch/2
  Sum9/1 -> Sum10/1
  Gain13/1 -> Multiport Switch/3
  Sum10/1 -> T_d/1  "T_d"
  Rate Transition/1 -> Sum9/1

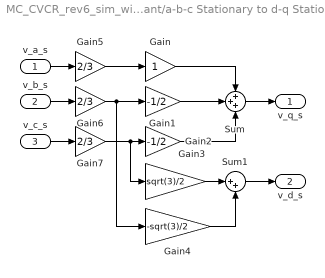
== system MC_CVCR_rev6_sim_withc_code_S_function_contplant/a-b-c Stationary to d-q Stationary ==
  v_a_s : Inport
  v_b_s : Inport  Port=2
  v_c_s : Inport  Port=3
  Gain : Gain
  Gain1 : Gain  Gain=-1/2
  Gain2 : Gain  Gain=-1/2
  Gain3 : Gain  Gain=sqrt(3)/2
  Gain4 : Gain  Gain=-sqrt(3)/2
  Gain5 : Gain  Gain=2/3
  Gain6 : Gain  Gain=2/3
  Gain7 : Gain  Gain=2/3
  Sum : Sum  Inputs=+++
  Sum1 : Sum  Inputs=|++
  v_q_s : Outport
  v_d_s : Outport  Port=2
  wires:
  v_b_s/1 -> Gain6/1
  v_a_s/1 -> Gain5/1
  Gain3/1 -> Sum1/1
  Gain4/1 -> Sum1/2
  Gain1/1 -> Sum/2
  Gain/1 -> Sum/1
  Gain2/1 -> Sum/3
  Sum/1 -> v_q_s/1
  Sum1/1 -> v_d_s/1
  v_c_s/1 -> Gain7/1
  Gain5/1 -> Gain/1
  Gain6/1 -> Gain4/1, Gain1/1
  Gain7/1 -> Gain3/1, Gain2/1

== system MC_CVCR_rev6_sim_withc_code_S_function_contplant/d-q Rotor to d-q Stationary ==
  v_q_e_star : Inport
  v_d_e_star : Inport  Port=2
  theta_re : Inport  Port=3
  Product{1..4} (4 alike) : Product
  Sum : Sum  Inputs=|++
  Sum1 : Sum  Inputs=|-+
  Trigonometric Function : Trigonometry
  Trigonometric Function1 : Trigonometry  Operator=cos
  v_q_s_star : Outport
  v_d_s_star : Outport  Port=2
  wires:
  v_q_e_star/1 -> Product3/1, Product1/1
  Trigonometric Function1/1 -> Product4/2, Product1/2
  v_d_e_star/1 -> Product2/1, Product4/1
  Trigonometric Function/1 -> Product3/2, Product2/2
  Product1/1 -> Sum/1
  Product2/1 -> Sum/2
  Product3/1 -> Sum1/1
  Product4/1 -> Sum1/2
  Sum/1 -> v_q_s_star/1
  Sum1/1 -> v_d_s_star/1
  theta_re/1 -> Trigonometric Function1/1, Trigonometric Function/1

== system MC_CVCR_rev6_sim_withc_code_S_function_contplant/d-q Rotor to a-b-c Stationary ==
  i_q_e : Inport
  i_d_e : Inport  Port=2
  theta : Inport  Port=3
  d-q Rotor to d-q Stationary : Subsystem
  d-q Stationary to a-b-c Stationary : Subsystem
  i_as : Outport
  i_bs : Outport  Port=2
  i_cs : Outport  Port=3
  wires:
  d-q Rotor to d-q Stationary/2(i_d_s) -> d-q Stationary to a-b-c Stationary/2(i_d_s)
  d-q Rotor to d-q Stationary/1(i_q_s) -> d-q Stationary to a-b-c Stationary/1(i_q_s)
  d-q Stationary to a-b-c Stationary/1(i_as) -> i_as/1
  d-q Stationary to a-b-c Stationary/2(i_bs) -> i_bs/1
  d-q Stationary to a-b-c Stationary/3(i_cs) -> i_cs/1
  i_d_e/1 -> d-q Rotor to d-q Stationary/2(i_d_e)  "i_d_e"
  i_q_e/1 -> d-q Rotor to d-q Stationary/1(i_q_e)  "i_q_e"
  theta/1 -> d-q Rotor to d-q Stationary/3(theta)  "theta"

== system MC_CVCR_rev6_sim_withc_code_S_function_contplant/d-q Stationary to a-b-c Stationary ==
  v_q_s : Inport
  v_d_s : Inport  Port=2
  Gain : Gain
  Gain1 : Gain  Gain=-1/2
  Gain2 : Gain  Gain=-sqrt(3)/2
  Gain3 : Gain  Gain=-1/2
  Gain4 : Gain  Gain=sqrt(3)/2
  Sum1 : Sum  Inputs=|++
  Sum2 : Sum  Inputs=|++
  v_a_s_star : Outport
  v_b_s_star : Outport  Port=2
  v_c_s_star : Outport  Port=3
  wires:
  v_q_s/1 -> Gain/1, Gain3/1, Gain1/1
  Gain1/1 -> Sum1/1
  Gain/1 -> v_a_s_star/1
  v_d_s/1 -> Gain4/1, Gain2/1
  Gain2/1 -> Sum1/2
  Gain3/1 -> Sum2/1
  Gain4/1 -> Sum2/2
  Sum1/1 -> v_b_s_star/1
  Sum2/1 -> v_c_s_star/1

== system MC_CVCR_rev6_sim_withc_code_S_function_contplant/d-q Stationary to d-q Rotor ==
  v_q_s : Inport
  v_d_s : Inport  Port=2
  theta_re : Inport  Port=3
  Product{1..4} (4 alike) : Product
  Sum : Sum  Inputs=|+-
  Sum1 : Sum  Inputs=|++
  Trigonometric Function : Trigonometry
  Trigonometric Function1 : Trigonometry  Operator=cos
  v_q_e : Outport
  v_d_e : Outport  Port=2
  wires:
  v_q_s/1 -> Product1/1, Product3/1
  theta_re/1 -> Trigonometric Function/1, Trigonometric Function1/1
  v_d_s/1 -> Product2/1, Product4/1
  Trigonometric Function/1 -> Product3/2, Product2/2
  Product1/1 -> Sum/1
  Product2/1 -> Sum/2
  Product3/1 -> Sum1/1
  Product4/1 -> Sum1/2
  Sum/1 -> v_q_e/1
  Sum1/1 -> v_d_e/1
  Trigonometric Function1/1 -> Product1/2, Product4/2

== system MC_CVCR_rev6_sim_withc_code_S_function_contplant/Complex Vector Current Regulator/Time weighted accum with saturation ==
  iqs_error : Inport
  Saturation : Saturate  UpperLimit=inf  LowerLimit=-inf
  Sum2 : Sum  Priority=1  Inputs=|++
  Unit Delay : UnitDelay  SampleTime=-1
  Velocity4 : Gain  Gain=T_s  SampleTime=T_s
  iqs_accum : Outport
  wires:
  Velocity4/1 -> Sum2/1
  Sum2/1 -> Saturation/1
  iqs_error/1 -> Velocity4/1
  Saturation/1 -> iqs_accum/1, Unit Delay/1
  Unit Delay/1 -> Sum2/2

== system MC_CVCR_rev6_sim_withc_code_S_function_contplant/Complex Vector Current Regulator/Time weighted accum with saturation1 ==
  iqs_error : Inport
  Saturation : Saturate  UpperLimit=inf  LowerLimit=-inf
  Sum2 : Sum  Priority=1  Inputs=|++
  Unit Delay : UnitDelay  SampleTime=-1
  Velocity4 : Gain  Gain=T_s  SampleTime=T_s
  iqs_accum : Outport
  wires:
  Velocity4/1 -> Sum2/1
  Sum2/1 -> Saturation/1
  iqs_error/1 -> Velocity4/1
  Saturation/1 -> iqs_accum/1, Unit Delay/1
  Unit Delay/1 -> Sum2/2

== system MC_CVCR_rev6_sim_withc_code_S_function_contplant/Motion Controller/TWA w// Sat ==
  error : Inport
  Saturation : Saturate  UpperLimit=inf  LowerLimit=-inf
  Scope : Scope
  Scope1 : Scope
  Sum2 : Sum  Priority=1  Inputs=|++
  Unit Delay : UnitDelay  SampleTime=-1
  accum : Outport
  wires:
  error/1 -> Sum2/1
  Saturation/1 -> Scope1/1, accum/1, Unit Delay/1
  Unit Delay/1 -> Sum2/2
  Sum2/1 -> Scope/1, Saturation/1

== system MC_CVCR_rev6_sim_withc_code_S_function_contplant/Motion Controller/TWA w// Sat1 ==
  error : Inport
  Saturation : Saturate  UpperLimit=inf  LowerLimit=-inf
  Sum2 : Sum  Priority=1  Inputs=|++
  Unit Delay : UnitDelay  SampleTime=-1
  accum : Outport
  wires:
  error/1 -> Sum2/1
  Sum2/1 -> Saturation/1
  Saturation/1 -> accum/1, Unit Delay/1
  Unit Delay/1 -> Sum2/2

== system MC_CVCR_rev6_sim_withc_code_S_function_contplant/Motion Observer/TWA w// Sat ==
  error : Inport
  Saturation : Saturate  UpperLimit=inf  LowerLimit=-inf
  Scope : Scope
  Scope1 : Scope
  Sum2 : Sum  Priority=1  Inputs=|++
  Unit Delay : UnitDelay  SampleTime=-1
  accum : Outport
  wires:
  error/1 -> Sum2/1
  Saturation/1 -> Scope1/1, accum/1, Unit Delay/1
  Unit Delay/1 -> Sum2/2
  Sum2/1 -> Scope/1, Saturation/1

== system MC_CVCR_rev6_sim_withc_code_S_function_contplant/Motion Observer/TWA w// Sat1 ==
  error : Inport
  Saturation : Saturate  UpperLimit=inf  LowerLimit=-inf
  Sum2 : Sum  Priority=1  Inputs=|++
  Unit Delay : UnitDelay  SampleTime=-1
  accum : Outport
  wires:
  error/1 -> Sum2/1
  Sum2/1 -> Saturation/1
  Saturation/1 -> accum/1, Unit Delay/1
  Unit Delay/1 -> Sum2/2

== system MC_CVCR_rev6_sim_withc_code_S_function_contplant/SIL/AB->ABC ==
  AB : Inport
  Mux2 : Mux  Inputs=3
  a : Fcn  Expr=u[1]
  b : Fcn  Expr=(-u[1]+sqrt(3)*u[2])/2
  c : Fcn  Expr=(-u[1]-sqrt(3)*u[2])/2
  ABC : Outport
  wires:
  Mux2/1 -> ABC/1
  b/1 -> Mux2/2
  c/1 -> Mux2/3
  AB/1 -> b/1, a/1, c/1
  a/1 -> Mux2/1

== system MC_CVCR_rev6_sim_withc_code_S_function_contplant/SIL/ABC-AB ==
  ABC : Inport
  Mux2 : Mux  Inputs=2
  a : Fcn  Expr=2/3*(u[1] -0.5*u[2] - 0.5*u[3])
  b : Fcn  Expr=2/3*(0 +sqrt(3)/2*u[2] - sqrt(3)/2*u[3])
  AB : Outport
  wires:
  Mux2/1 -> AB/1
  b/1 -> Mux2/2
  ABC/1 -> b/1, a/1
  a/1 -> Mux2/1

== system MC_CVCR_rev6_sim_withc_code_S_function_contplant/d-q Rotor to a-b-c Stationary/d-q Rotor to d-q Stationary ==
  i_q_e : Inport
  i_d_e : Inport  Port=2
  theta : Inport  Port=3
  Product{1..4} (4 alike) : Product
  Sum : Sum  Inputs=|++
  Sum1 : Sum  Inputs=|-+
  Trigonometric Function : Trigonometry
  Trigonometric Function1 : Trigonometry  Operator=cos
  i_q_s : Outport
  i_d_s : Outport  Port=2
  wires:
  i_q_e/1 -> Product1/1, Product3/1
  i_d_e/1 -> Product4/1, Product2/1
  Trigonometric Function/1 -> Product3/2, Product2/2
  Product1/1 -> Sum/1
  Product2/1 -> Sum/2
  Product3/1 -> Sum1/1
  Product4/1 -> Sum1/2
  Sum/1 -> i_q_s/1
  Sum1/1 -> i_d_s/1
  theta/1 -> Trigonometric Function/1, Trigonometric Function1/1
  Trigonometric Function1/1 -> Product4/2, Product1/2

== system MC_CVCR_rev6_sim_withc_code_S_function_contplant/d-q Rotor to a-b-c Stationary/d-q Stationary to a-b-c Stationary ==
  i_q_s : Inport
  i_d_s : Inport  Port=2
  Gain : Gain
  Gain1 : Gain  Gain=-1/2
  Gain2 : Gain  Gain=-sqrt(3)/2
  Gain3 : Gain  Gain=-1/2
  Gain4 : Gain  Gain=sqrt(3)/2
  Sum1 : Sum  Inputs=|++
  Sum2 : Sum  Inputs=|++
  i_as : Outport
  i_bs : Outport  Port=2
  i_cs : Outport  Port=3
  wires:
  i_q_s/1 -> Gain/1, Gain3/1, Gain1/1
  Gain1/1 -> Sum1/1
  Gain/1 -> i_as/1
  i_d_s/1 -> Gain4/1, Gain2/1
  Gain2/1 -> Sum1/2
  Gain3/1 -> Sum2/1
  Gain4/1 -> Sum2/2
  Sum1/1 -> i_bs/1
  Sum2/1 -> i_cs/1
